simulink model "p_i_d_controller"  (R2017b)
settings: Solver=VariableStepAuto  StartTime=0.0  StopTime=10  RelTol=1e-3
libraries: simulink x1
settings Model: Creator=Alec  LastModifiedBy=Alec

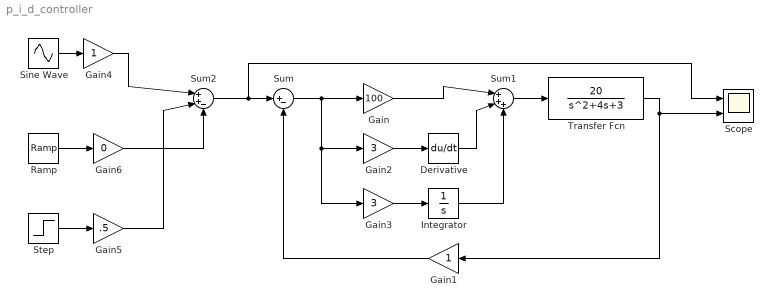
== system p_i_d_controller ==
  Derivative : Derivative
  Gain : Gain  Gain=100
  Gain1 : Gain
  Gain2 : Gain  Gain=3
  Gain3 : Gain  Gain=3
  Gain4 : Gain
  Gain5 : Gain  Gain=.5
  Gain6 : Gain  Gain=0
  Integrator : Integrator
  Ramp : simulink/Sources/Ramp  slope=.1  start=0  X0=0
  Scope : Scope  NumInputPorts=2
  Sine Wave : Sin  Amplitude=.25  Phase=pi/2  SampleTime=0
  Step : Step  SampleTime=0
  Sum : Sum  Inputs=|+-
  Sum1 : Sum  Inputs=|+++
  Sum2 : Sum  Inputs=|++-
  Transfer Fcn : TransferFcn  Numerator=[20]  Denominator=[1 4 3]
  wires:
  Sum/1 -> Gain/1, Gain2/1, Gain3/1
  Gain1/1 -> Sum/2
  Gain2/1 -> Derivative/1
  Sum1/1 -> Transfer Fcn/1
  Gain/1 -> Sum1/1
  Transfer Fcn/1 -> Scope/2, Gain1/1
  Derivative/1 -> Sum1/2
  Gain3/1 -> Integrator/1
  Integrator/1 -> Sum1/3
  Ramp/1 -> Gain6/1
  Step/1 -> Gain5/1
  Sine Wave/1 -> Gain4/1
  Sum2/1 -> Scope/1, Sum/1
  Gain6/1 -> Sum2/3
  Gain4/1 -> Sum2/1
  Gain5/1 -> Sum2/2
